simulink model "C_elegans"  (Simulink 7.0)
settings: Solver=ode45  StartTime=0.0  StopTime=10.0  FixedStep=1e-3
undefined symbols (not defined in the file or in its folder): A_n, beta_0M, beta_D, beta_L, c_par, c_per, d_Time, End_Time, eps_hys, F_max_i, G_SR_n, gamma_iD, gamma_iV, I_AVB_D, I_AVB_V, kappa_0M, kappa_D, kappa_L, L_0D_i, L_0L_i, L_min_i, lambda_i, M_num, N_out, N_SR, not_w_NMJ, phi0_vec, R_i, Ri_c_per, S0_nk, tau_M, w_D, w_NMJ, w_V, X_com0
libraries: simulink x1
settings Model: Creator=KRproject  LastModifiedBy=KRproject  SimulationMode=rapid-accelerator
settings OptimizationCC: InlineParams=on  SimCompilerOptimization=On

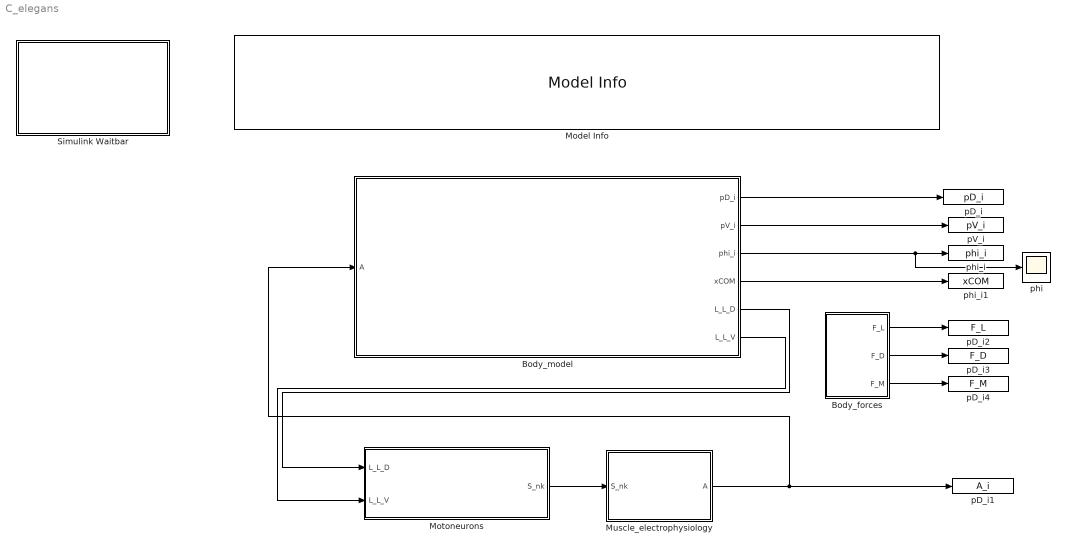
== system C_elegans ==
  Body_forces : Subsystem
  Body_model : Subsystem
      mask Display:
      | image(imread('./pictures/Body_model.png'))
      | port_label('input', 1, 'A')
      | port_label('output', 1, 'pD_i')
      | port_label('output', 2, 'pV_i')
      | port_label('output', 3, 'phi_i')
      | port_label('output', 4, 'xCOM')
      | port_label('output', 5, 'L_L_D')
      | port_label('output', 6, 'L_L_V')
  Model Info : simulink/Model-Wide Utilities/Model Info  SystemSampleTime=-1  InitialBlockCM=None  BlockCM=None  Frame=on  DisplayStringWithTags=|  HorizontalTextAlignment=Center  LeftAlignmentValue=0.5  SourceBlockDiagram=C_elegans  TagMaxNumber=20
      | March 2012
      | C elegans integrated model
      | 
      | ' J. Boyleet al., Gait modulation in C.elegans: an integrated neuromechanical model, Frontiers in Computational Neuroscience, 2012. '
  Motoneurons : Subsystem
  Muscle_electrophysiology : Subsystem
  Simulink Waitbar : Subsystem
      mask Display: image(imread('./pictures/sim_wait.png'))
  pD_i : ToWorkspace  VariableName=pD_i  SampleTime=d_Time  SaveFormat=Array
  pD_i1 : ToWorkspace  VariableName=A_i  SampleTime=d_Time  SaveFormat=Array
  pD_i2 : ToWorkspace  VariableName=F_L  SampleTime=d_Time  SaveFormat=Array
  pD_i3 : ToWorkspace  VariableName=F_D  SampleTime=d_Time  SaveFormat=Array
  pD_i4 : ToWorkspace  VariableName=F_M  SampleTime=d_Time  SaveFormat=Array
  pV_i : ToWorkspace  VariableName=pV_i  SampleTime=d_Time  SaveFormat=Array
  phi : Scope
      settings: TimeRange=10  YMin=-0.75  YMax=3.75
  phi_i : ToWorkspace  VariableName=phi_i  SampleTime=d_Time  SaveFormat=Array
  phi_i1 : ToWorkspace  VariableName=xCOM  SampleTime=d_Time  SaveFormat=Array
  wires:
  Body_model/1(pD_i) -> pD_i/1
  Body_model/2(pV_i) -> pV_i/1
  Body_model/3(phi_i) -> phi_i/1, phi/1
  Body_model/5(L_L_D) -> Motoneurons/1(L_L_D)
  Body_model/6(L_L_V) -> Motoneurons/2(L_L_V)
  Motoneurons/1(S_nk) -> Muscle_electrophysiology/1(S_nk)
  Muscle_electrophysiology/1(A) -> pD_i1/1, Body_model/1(A)
  Body_model/4(xCOM) -> phi_i1/1
  Body_forces/1(F_L) -> pD_i2/1
  Body_forces/2(F_D) -> pD_i3/1
  Body_forces/3(F_M) -> pD_i4/1

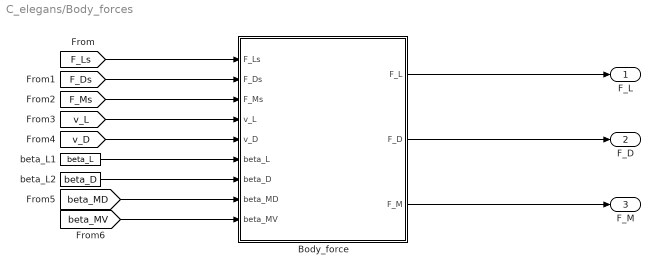
== system C_elegans/Body_forces ==
  Body_force : Stateflow chart
  beta_L1 : Constant  Value=beta_L  OutDataType=sfix(16)  OutScaling=2^0
  beta_L2 : Constant  Value=beta_D  OutDataType=sfix(16)  OutScaling=2^0
  F_L : Outport
  F_D : Outport  Port=2
  F_M : Outport  Port=3
  wires:
  [F_Ls] -> Body_force/1(F_Ls)
  [F_Ds] -> Body_force/2(F_Ds)
  [F_Ms] -> Body_force/3(F_Ms)
  [v_L] -> Body_force/4(v_L)
  [v_D] -> Body_force/5(v_D)
  beta_L1/1 -> Body_force/6(beta_L)
  beta_L2/1 -> Body_force/7(beta_D)
  [beta_MD] -> Body_force/8(beta_MD)
  [beta_MV] -> Body_force/9(beta_MV)
  Body_force/1(F_L) -> F_L/1
  Body_force/2(F_D) -> F_D/1
  Body_force/3(F_M) -> F_M/1

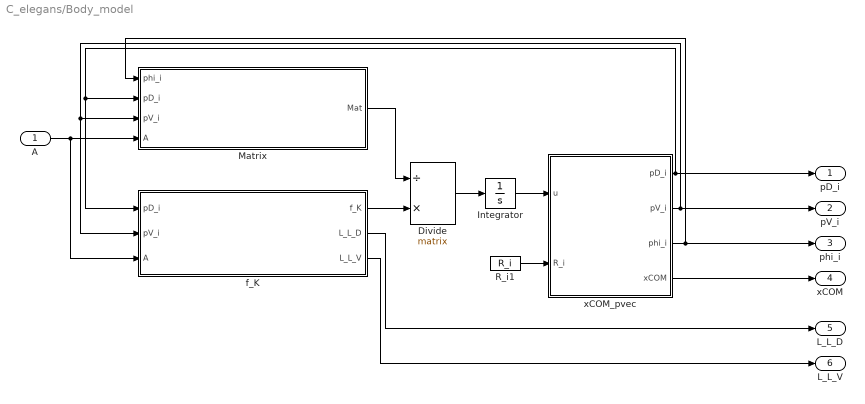
== system C_elegans/Body_model ==
  A : Inport
  Divide : Product  Inputs=/*  Multiplication=Matrix(*)  OutDataType=sfix(16)  OutScaling=2^-10
  Integrator : Integrator  InitialCondition=[ X_com0; phi0_vec]
  Matrix : Subsystem
      mask Display:
      | image(imread('./pictures/Matrix.png'))
      | 
      | port_label('output', 1, 'Mat')
      | port_label('input', 1, 'phi_i')
      | port_label('input', 2, 'pD_i')
      | port_label('input', 3, 'pV_i')
      | port_label('input', 4, 'A')
  R_i1 : Constant  Value=R_i  OutDataType=sfix(16)  OutScaling=2^0
  f_K : Subsystem
      mask Display:
      | image(imread('./pictures/vect.png'))
      | 
      | port_label('output', 1, 'f_K')
      | port_label('output', 2, 'L_L_D')
      | port_label('output', 3, 'L_L_V')
      | 
      | port_label('input', 1, 'pD_i')
      | port_label('input', 2, 'pV_i')
      | port_label('input', 3, 'A')
  xCOM_pvec : Stateflow chart
  pD_i : Outport
  pV_i : Outport  Port=2
  phi_i : Outport  Port=3
  xCOM : Outport  Port=4
  L_L_D : Outport  Port=5
  L_L_V : Outport  Port=6
  wires:
  A/1 -> Matrix/4(A), f_K/3(A)
  Matrix/1(Mat) -> Divide/1
  f_K/1(f_K) -> Divide/2
  Integrator/1 -> xCOM_pvec/1(u)
  R_i1/1 -> xCOM_pvec/2(R_i)
  xCOM_pvec/1(pD_i) -> Matrix/2(pD_i), f_K/1(pD_i), pD_i/1
  xCOM_pvec/2(pV_i) -> Matrix/3(pV_i), f_K/2(pV_i), pV_i/1
  xCOM_pvec/3(phi_i) -> Matrix/1(phi_i), phi_i/1
  f_K/2(L_L_D) -> L_L_D/1
  f_K/3(L_L_V) -> L_L_V/1
  xCOM_pvec/4(xCOM) -> xCOM/1
  Divide/1 -> Integrator/1

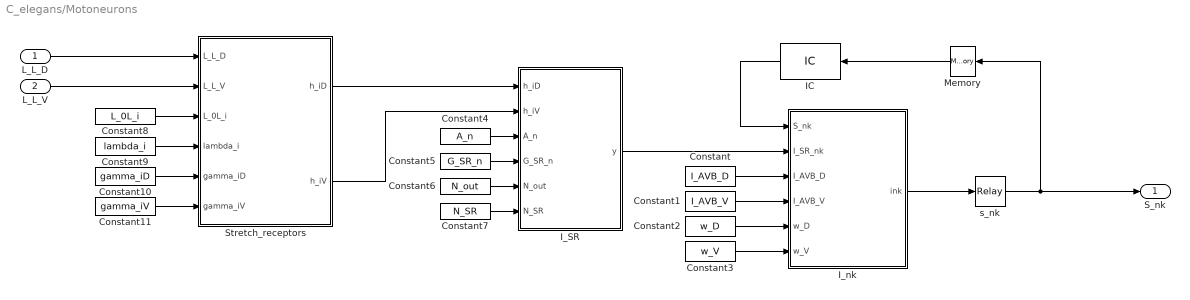
== system C_elegans/Motoneurons ==
  L_L_D : Inport
  L_L_V : Inport  Port=2
  Constant : Constant  Value=I_AVB_D  OutDataType=sfix(16)  OutScaling=2^0
  Constant1 : Constant  Value=I_AVB_V  OutDataType=sfix(16)  OutScaling=2^0
  Constant10 : Constant  Value=gamma_iD  OutDataType=sfix(16)  OutScaling=2^0
  Constant11 : Constant  Value=gamma_iV  OutDataType=sfix(16)  OutScaling=2^0
  Constant2 : Constant  Value=w_D  OutDataType=sfix(16)  OutScaling=2^0
  Constant3 : Constant  Value=w_V  OutDataType=sfix(16)  OutScaling=2^0
  Constant4 : Constant  Value=A_n  OutDataType=sfix(16)  OutScaling=2^0
  Constant5 : Constant  Value=G_SR_n  OutDataType=sfix(16)  OutScaling=2^0
  Constant6 : Constant  Value=N_out  OutDataType=sfix(16)  OutScaling=2^0
  Constant7 : Constant  Value=N_SR  OutDataType=sfix(16)  OutScaling=2^0
  Constant8 : Constant  Value=L_0L_i  OutDataType=sfix(16)  OutScaling=2^0
  Constant9 : Constant  Value=lambda_i  OutDataType=sfix(16)  OutScaling=2^0
  IC : InitialCondition  Orientation=left  Value=S0_nk
  I_SR : Stateflow chart
  I_nk : Stateflow chart
  Memory : Memory  Orientation=left
  Stretch_receptors : Stateflow chart
  s_nk : Relay  OnSwitchValue=0.5*(1 + eps_hys)  OffSwitchValue=0.5*(1 - eps_hys)  OutDataType=sfix(16)  OutScaling=2^0
  S_nk : Outport
  wires:
  s_nk/1 -> S_nk/1, Memory/1
  I_nk/1(ink) -> s_nk/1
  Constant/1 -> I_nk/3(I_AVB_D)
  Constant1/1 -> I_nk/4(I_AVB_V)
  Constant2/1 -> I_nk/5(w_D)
  Constant3/1 -> I_nk/6(w_V)
  IC/1 -> I_nk/1(S_nk)
  I_SR/1(y) -> I_nk/2(I_SR_nk)
  Constant4/1 -> I_SR/3(A_n)
  Constant5/1 -> I_SR/4(G_SR_n)
  Constant6/1 -> I_SR/5(N_out)
  Constant7/1 -> I_SR/6(N_SR)
  Stretch_receptors/1(h_iD) -> I_SR/1(h_iD)
  Stretch_receptors/2(h_iV) -> I_SR/2(h_iV)
  Constant8/1 -> Stretch_receptors/3(L_0L_i)
  Constant9/1 -> Stretch_receptors/4(lambda_i)
  Constant10/1 -> Stretch_receptors/5(gamma_iD)
  Constant11/1 -> Stretch_receptors/6(gamma_iV)
  L_L_D/1 -> Stretch_receptors/1(L_L_D)
  L_L_V/1 -> Stretch_receptors/2(L_L_V)
  Memory/1 -> IC/1

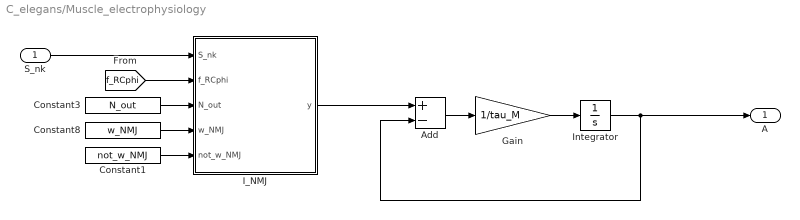
== system C_elegans/Muscle_electrophysiology ==
  S_nk : Inport
  Add : Sum  Inputs=+-  OutDataType=sfix(16)  OutScaling=2^-10
  Constant1 : Constant  Value=not_w_NMJ  OutDataType=sfix(16)  OutScaling=2^0
  Constant3 : Constant  Value=N_out  OutDataType=sfix(16)  OutScaling=2^0
  Constant8 : Constant  Value=w_NMJ  OutDataType=sfix(16)  OutScaling=2^0
  Gain : Gain  Gain=1/tau_M  ParameterDataType=sfix(16)  ParameterScaling=2^0  OutDataType=sfix(16)  OutScaling=2^0
  I_NMJ : Stateflow chart
  Integrator : Integrator  InitialCondition=zeros(2*M_num,1)
  A : Outport
  wires:
  Constant1/1 -> I_NMJ/5(not_w_NMJ)
  Constant8/1 -> I_NMJ/4(w_NMJ)
  I_NMJ/1(y) -> Add/1
  Add/1 -> Gain/1
  Integrator/1 -> Add/2, A/1
  Gain/1 -> Integrator/1
  Constant3/1 -> I_NMJ/3(N_out)
  [f_RCphi] -> I_NMJ/2(f_RCphi)
  S_nk/1 -> I_NMJ/1(S_nk)

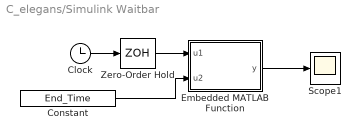
== system C_elegans/Simulink Waitbar ==
  Clock : Clock
  Constant : Constant  Value=End_Time  OutDataType=sfix(16)  OutScaling=2^0
  Embedded MATLAB Function : Stateflow chart
  Scope1 : Scope
      settings: YMin=1  YMax=1  SaveName=ScopeData2
  Zero-Order Hold : ZeroOrderHold
  wires:
  Clock/1 -> Zero-Order Hold/1
  Constant/1 -> Embedded MATLAB Function/2(u2)
  Embedded MATLAB Function/1(y) -> Scope1/1
  Zero-Order Hold/1 -> Embedded MATLAB Function/1(u1)

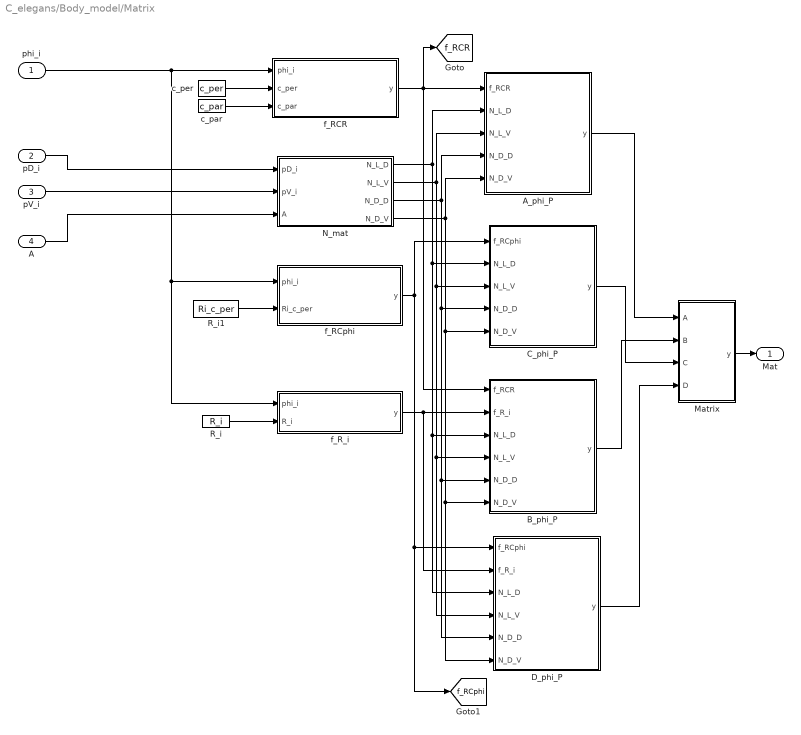
== system C_elegans/Body_model/Matrix ==
  phi_i : Inport
  pD_i : Inport  Port=2
  pV_i : Inport  Port=3
  A : Inport  Port=4
  A_phi_P : Stateflow chart
  B_phi_P : Stateflow chart
  C_phi_P : Stateflow chart
  D_phi_P : Stateflow chart
  Matrix : Stateflow chart
  N_mat : Subsystem
  R_i : Constant  Value=R_i  OutDataType=sfix(16)  OutScaling=2^0
  R_i1 : Constant  Value=Ri_c_per  OutDataType=sfix(16)  OutScaling=2^0
  c_par : Constant  Value=c_par  OutDataType=sfix(16)  OutScaling=2^0
  c_per : Constant  Value=c_per  OutDataType=sfix(16)  OutScaling=2^0
  f_RCR : Stateflow chart
  f_RCphi : Stateflow chart
  f_R_i : Stateflow chart
  Mat : Outport
  tag scope: f_RCR=global, f_RCphi=global
  wires:
  c_per/1 -> f_RCR/2(c_per)
  c_par/1 -> f_RCR/3(c_par)
  f_RCR/1(y) -> A_phi_P/1(f_RCR), B_phi_P/1(f_RCR), [f_RCR]
  N_mat/1(N_L_D) -> A_phi_P/2(N_L_D), C_phi_P/2(N_L_D), B_phi_P/3(N_L_D), D_phi_P/3(N_L_D)
  N_mat/2(N_L_V) -> A_phi_P/3(N_L_V), C_phi_P/3(N_L_V), B_phi_P/4(N_L_V), D_phi_P/4(N_L_V)
  N_mat/3(N_D_D) -> A_phi_P/4(N_D_D), B_phi_P/5(N_D_D), D_phi_P/5(N_D_D), C_phi_P/4(N_D_D)
  N_mat/4(N_D_V) -> A_phi_P/5(N_D_V), B_phi_P/6(N_D_V), D_phi_P/6(N_D_V), C_phi_P/5(N_D_V)
  A_phi_P/1(y) -> Matrix/1(A)
  R_i/1 -> f_R_i/2(R_i)
  f_RCphi/1(y) -> C_phi_P/1(f_RCphi), D_phi_P/1(f_RCphi), [f_RCphi]
  f_R_i/1(y) -> B_phi_P/2(f_R_i), D_phi_P/2(f_R_i)
  C_phi_P/1(y) -> Matrix/3(C)
  B_phi_P/1(y) -> Matrix/2(B)
  D_phi_P/1(y) -> Matrix/4(D)
  phi_i/1 -> f_RCR/1(phi_i), f_R_i/1(phi_i), f_RCphi/1(phi_i)
  pD_i/1 -> N_mat/1(pD_i)
  pV_i/1 -> N_mat/2(pV_i)
  A/1 -> N_mat/3(A)
  Matrix/1(y) -> Mat/1
  R_i1/1 -> f_RCphi/2(Ri_c_per)

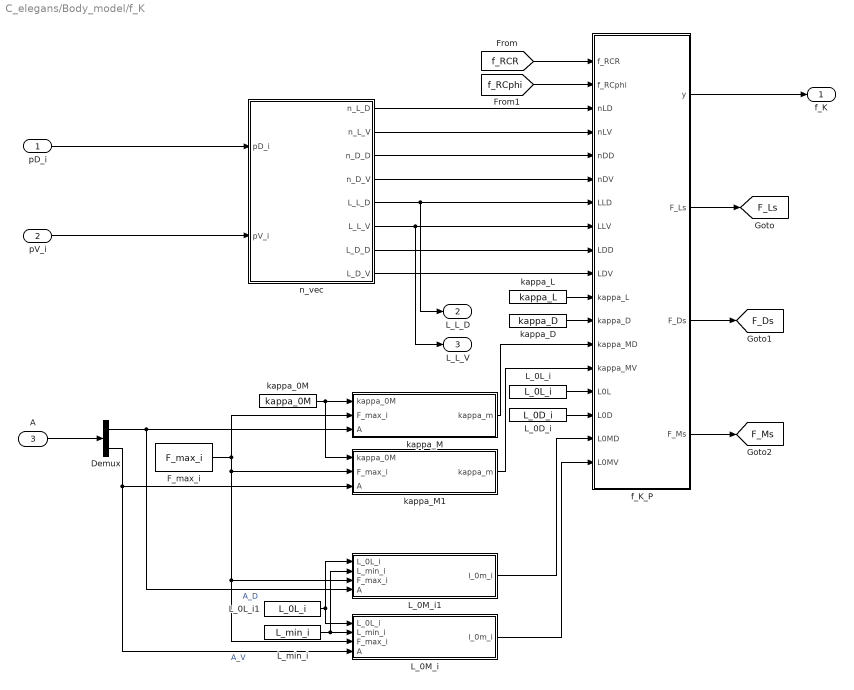
== system C_elegans/Body_model/f_K ==
  pD_i : Inport
  pV_i : Inport  Port=2
  A : Inport  Port=3
  Demux : Demux  Outputs=2
  F_max_i : Constant  Value=F_max_i  OutDataType=sfix(16)  OutScaling=2^0
  L_0D_i : Constant  Value=L_0D_i  OutDataType=sfix(16)  OutScaling=2^0
  L_0L_i : Constant  Value=L_0L_i  OutDataType=sfix(16)  OutScaling=2^0
  L_0L_i1 : Constant  Value=L_0L_i  OutDataType=sfix(16)  OutScaling=2^0
  L_0M_i : Stateflow chart
  L_0M_i1 : Stateflow chart
  L_min_i : Constant  Value=L_min_i  OutDataType=sfix(16)  OutScaling=2^0
  f_K_P : Stateflow chart
  kappa_0M : Constant  Value=kappa_0M  OutDataType=sfix(16)  OutScaling=2^0
  kappa_D : Constant  Value=kappa_D  OutDataType=sfix(16)  OutScaling=2^0
  kappa_L : Constant  Value=kappa_L  OutDataType=sfix(16)  OutScaling=2^0
  kappa_M : Stateflow chart
  kappa_M1 : Stateflow chart
  n_vec : Subsystem
  f_K : Outport
  L_L_D : Outport  Port=2
  L_L_V : Outport  Port=3
  tag scope: F_Ds=global, F_Ls=global, F_Ms=global
  wires:
  n_vec/1(n_L_D) -> f_K_P/3(nLD)
  n_vec/2(n_L_V) -> f_K_P/4(nLV)
  n_vec/3(n_D_D) -> f_K_P/5(nDD)
  n_vec/4(n_D_V) -> f_K_P/6(nDV)
  n_vec/5(L_L_D) -> f_K_P/7(LLD), L_L_D/1
  n_vec/6(L_L_V) -> f_K_P/8(LLV), L_L_V/1
  n_vec/7(L_D_D) -> f_K_P/9(LDD)
  n_vec/8(L_D_V) -> f_K_P/10(LDV)
  L_0L_i/1 -> f_K_P/15(L0L)
  kappa_L/1 -> f_K_P/11(kappa_L)
  L_0D_i/1 -> f_K_P/16(L0D)
  kappa_D/1 -> f_K_P/12(kappa_D)
  kappa_0M/1 -> kappa_M/1(kappa_0M), kappa_M1/1(kappa_0M)
  L_min_i/1 -> L_0M_i/2(L_min_i), L_0M_i1/2(L_min_i)
  F_max_i/1 -> kappa_M/2(F_max_i), kappa_M1/2(F_max_i), L_0M_i/3(F_max_i), L_0M_i1/3(F_max_i)
  kappa_M/1(kappa_m) -> f_K_P/13(kappa_MD)
  L_0M_i/1(l_0m_i) -> f_K_P/18(L0MV)
  pD_i/1 -> n_vec/1(pD_i)
  pV_i/1 -> n_vec/2(pV_i)
  f_K_P/1(y) -> f_K/1
  A/1 -> Demux/1
  Demux/1 -> kappa_M/3(A), L_0M_i1/4(A)  "A_D"
  Demux/2 -> L_0M_i/4(A), kappa_M1/3(A)  "A_V"
  kappa_M1/1(kappa_m) -> f_K_P/14(kappa_MV)
  L_0M_i1/1(l_0m_i) -> f_K_P/17(L0MD)
  L_0L_i1/1 -> L_0M_i/1(L_0L_i), L_0M_i1/1(L_0L_i)
  [f_RCR] -> f_K_P/1(f_RCR)
  [f_RCphi] -> f_K_P/2(f_RCphi)
  f_K_P/2(F_Ls) -> [F_Ls]
  f_K_P/3(F_Ds) -> [F_Ds]
  f_K_P/4(F_Ms) -> [F_Ms]

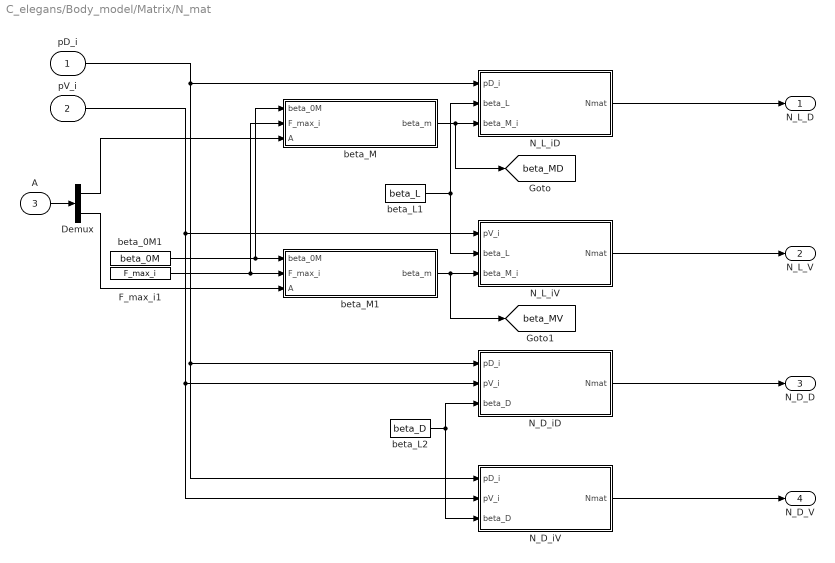
== system C_elegans/Body_model/Matrix/N_mat ==
  pD_i : Inport
  pV_i : Inport  Port=2
  A : Inport  Port=3
  Demux : Demux  Outputs=[M_num,M_num]
  F_max_i1 : Constant  Value=F_max_i  OutDataType=sfix(16)  OutScaling=2^0
  N_D_iD : Stateflow chart
  N_D_iV : Stateflow chart
  N_L_iD : Stateflow chart
  N_L_iV : Stateflow chart
  beta_0M1 : Constant  Value=beta_0M  OutDataType=sfix(16)  OutScaling=2^0
  beta_L1 : Constant  Value=beta_L  OutDataType=sfix(16)  OutScaling=2^0
  beta_L2 : Constant  Value=beta_D  OutDataType=sfix(16)  OutScaling=2^0
  beta_M : Stateflow chart
  beta_M1 : Stateflow chart
  N_L_D : Outport
  N_L_V : Outport  Port=2
  N_D_D : Outport  Port=3
  N_D_V : Outport  Port=4
  tag scope: beta_MD=global, beta_MV=global
  wires:
  beta_M/1(beta_m) -> N_L_iD/3(beta_M_i), [beta_MD]
  Demux/1 -> beta_M/3(A)
  beta_L1/1 -> N_L_iV/2(beta_L), N_L_iD/2(beta_L)
  beta_0M1/1 -> beta_M1/1(beta_0M), beta_M/1(beta_0M)
  F_max_i1/1 -> beta_M1/2(F_max_i), beta_M/2(F_max_i)
  beta_M1/1(beta_m) -> N_L_iV/3(beta_M_i), [beta_MV]
  Demux/2 -> beta_M1/3(A)
  beta_L2/1 -> N_D_iD/3(beta_D), N_D_iV/3(beta_D)
  pD_i/1 -> N_L_iD/1(pD_i), N_D_iD/1(pD_i), N_D_iV/1(pD_i)
  A/1 -> Demux/1
  pV_i/1 -> N_L_iV/1(pV_i), N_D_iD/2(pV_i), N_D_iV/2(pV_i)
  N_L_iD/1(Nmat) -> N_L_D/1
  N_L_iV/1(Nmat) -> N_L_V/1
  N_D_iD/1(Nmat) -> N_D_D/1
  N_D_iV/1(Nmat) -> N_D_V/1

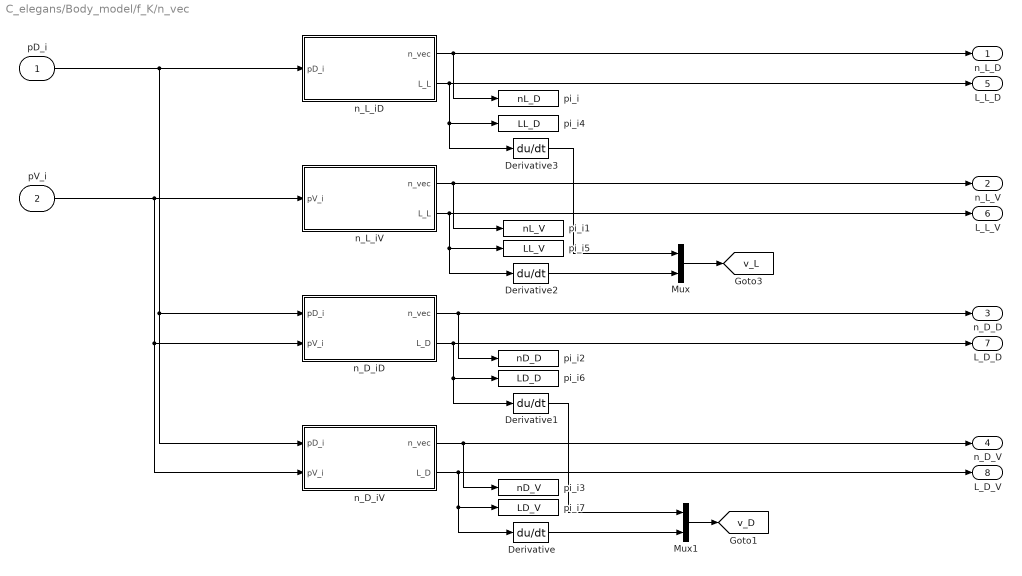
== system C_elegans/Body_model/f_K/n_vec ==
  pD_i : Inport
  pV_i : Inport  Port=2
  Derivative{,1..3} (4 alike) : Derivative
  Mux : Mux  Inputs=2
  Mux1 : Mux  Inputs=2
  n_D_iD : Stateflow chart
  n_D_iV : Stateflow chart
  n_L_iD : Stateflow chart
  n_L_iV : Stateflow chart
  pi_i : ToWorkspace  VariableName=nL_D  SampleTime=d_Time  SaveFormat=Array
  pi_i1 : ToWorkspace  VariableName=nL_V  SampleTime=d_Time  SaveFormat=Array
  pi_i2 : ToWorkspace  VariableName=nD_D  SampleTime=d_Time  SaveFormat=Array
  pi_i3 : ToWorkspace  VariableName=nD_V  SampleTime=d_Time  SaveFormat=Array
  pi_i4 : ToWorkspace  VariableName=LL_D  SampleTime=d_Time  SaveFormat=Array
  pi_i5 : ToWorkspace  VariableName=LL_V  SampleTime=d_Time  SaveFormat=Array
  pi_i6 : ToWorkspace  VariableName=LD_D  SampleTime=d_Time  SaveFormat=Array
  pi_i7 : ToWorkspace  VariableName=LD_V  SampleTime=d_Time  SaveFormat=Array
  n_L_D : Outport
  n_L_V : Outport  Port=2
  n_D_D : Outport  Port=3
  n_D_V : Outport  Port=4
  L_L_D : Outport  Port=5
  L_L_V : Outport  Port=6
  L_D_D : Outport  Port=7
  L_D_V : Outport  Port=8
  tag scope: v_D=global, v_L=global
  wires:
  pD_i/1 -> n_L_iD/1(pD_i), n_D_iD/1(pD_i), n_D_iV/1(pD_i)
  pV_i/1 -> n_L_iV/1(pV_i), n_D_iD/2(pV_i), n_D_iV/2(pV_i)
  n_L_iD/1(n_vec) -> n_L_D/1, pi_i/1
  n_L_iV/1(n_vec) -> n_L_V/1, pi_i1/1
  n_D_iD/1(n_vec) -> n_D_D/1, pi_i2/1
  n_D_iV/1(n_vec) -> n_D_V/1, pi_i3/1
  n_L_iD/2(L_L) -> L_L_D/1, pi_i4/1, Derivative3/1
  n_L_iV/2(L_L) -> L_L_V/1, pi_i5/1, Derivative2/1
  n_D_iD/2(L_D) -> L_D_D/1, pi_i6/1, Derivative1/1
  n_D_iV/2(L_D) -> L_D_V/1, pi_i7/1, Derivative/1
  Mux1/1 -> [v_D]
  Mux/1 -> [v_L]
  Derivative/1 -> Mux1/2
  Derivative2/1 -> Mux/2
  Derivative3/1 -> Mux/1
  Derivative1/1 -> Mux1/1

== matlab function Body_model/f_K/kappa_M1 ==
  data: kappa_0M input inherited; kappa_m output inherited; F_max_i input inherited; A input inherited
function kappa_m = kappa_M( kappa_0M, F_max_i, A)
% This block supports the Embedded MATLAB subset.
% See the help menu for details. 

sig_A = A.*( 0 < A & A < 1) + (1 <= A);

kappa_m = kappa_0M.*F_max_i.*sig_A;

== matlab function Body_model/f_K/L_0M_i1 ==
  data: L_0L_i input inherited; L_min_i input inherited; l_0m_i output inherited; F_max_i input inherited; A input inherited
function l_0m_i = L_0M_i( L_0L_i, L_min_i, F_max_i, A)
% This block supports the Embedded MATLAB subset.
% See the help menu for details. 

sig_A = A.*( 0 < A & A < 1) + (1 <= A);

l_0m_i = L_0L_i - F_max_i.*sig_A.*(L_0L_i - L_min_i);

== matlab function Motoneurons/I_nk ==
  data: S_nk input inherited; I_SR_nk input inherited; ink output inherited; I_AVB_D input inherited; I_AVB_V input inherited; w_D input inherited; w_V input inherited
function ink = I_nk( S_nk, I_SR_nk, I_AVB_D, I_AVB_V, w_D, w_V)
% This block supports the Embedded MATLAB subset.
% See the help menu for details. 

N_num = length( S_nk)/2;

S_nD = S_nk(1:N_num);
S_nV = S_nk(N_num+1:end);

I_SR_nD = I_SR_nk(1:N_num);
I_SR_nV = I_SR_nk(N_num+1:end);


ink = 0*S_nk;
ink(1:N_num) = I_AVB_D + I_SR_nD + w_D*S_nV;
ink(N_num+1:end) = I_AVB_V + I_SR_nV + w_V*S_nD;

== matlab function Motoneurons/I_SR ==
  data: h_iD input inherited; h_iV input inherited; y output inherited; A_n input inherited; G_SR_n input inherited; N_out input inherited; N_SR input inherited
function y = I_SR( h_iD, h_iV, A_n, G_SR_n, N_out, N_SR)
% This block supports the Embedded MATLAB subset.
% See the help menu for details. 

N_num = length( A_n);
M_num = length( h_iD);

H_iD = 0*A_n;
H_iV = 0*A_n;
for n = 1:N_num 
    
    s_end = min( M_num, N_SR + (n - 1)*N_out);
    for m = 1:M_num
        
        H_iD(n) = H_iD(n) + h_iD(m).*( (n-1)*N_out+1 <= m & m <= s_end);
        H_iV(n) = H_iV(n) + h_iV(m).*( (n-1)*N_out+1 <= m & m <= s_end);
    end
end

y = repmat( A_n.*G_SR_n, 2, 1).*[ H_iD; 
                                  H_iV];

== matlab function Motoneurons/Stretch_receptors ==
  data: L_L_D input inherited; h_iD output inherited; L_L_V input inherited; L_0L_i input inherited; lambda_i input inherited; gamma_iD input inherited; gamma_iV input inherited; h_iV output inherited
function [h_iD,h_iV] = h_ik( L_L_D, L_L_V, L_0L_i, lambda_i, gamma_iD, gamma_iV)
% This block supports the Embedded MATLAB subset.
% See the help menu for details. 

h_iD = lambda_i.*( gamma_iD(1)*(L_L_D - L_0L_i)./L_0L_i.*(L_L_D > L_0L_i) ...
                  + gamma_iD(2)*(L_L_D - L_0L_i)./L_0L_i.*(L_L_D <= L_0L_i) );
h_iV = lambda_i*gamma_iV.*(L_L_V - L_0L_i)./L_0L_i;

== matlab function Simulink Waitbar/Embedded MATLAB Function ==
  data: u1 input inherited; y output inherited; u2 input inherited
function y = fcn(u1, u2)
% This block supports an embeddable subset of the MATLAB language.
% See the help menu for details. 

eml.extrinsic('waitbar')

waitbar(u1/u2)
y = 1;

== matlab function Muscle_electrophysiology/I_NMJ ==
  data: S_nk input inherited; f_RCphi input inherited; N_out input inherited; y output inherited; w_NMJ input inherited; not_w_NMJ input inherited
function y = I_NMJ( S_nk, f_RCphi, N_out, w_NMJ, not_w_NMJ)
% This block supports the Embedded MATLAB subset.
% See the help menu for details. 

N_num = length( S_nk)/2;

S_nD = S_nk(1:N_num);
S_nV = S_nk(N_num+1:end);

M_num = size( f_RCphi, 1) - 1;
zero_vec = 0*f_RCphi(1:end-1,1);
i_NMJ_D = zero_vec;
i_NMJ_V = zero_vec;
for i=1:M_num
    
    n = ceil( i/N_out);
    
    i_NMJ_D(i) = w_NMJ(n)*S_nD(n) + not_w_NMJ(n)*S_nV(n);
    i_NMJ_V(i) = w_NMJ(n)*S_nV(n) + not_w_NMJ(n)*S_nD(n);
end

y = [ i_NMJ_D;
      i_NMJ_V];

== matlab function Body_forces/Body_force ==
  data: F_Ls input inherited; F_L output inherited; F_Ds input inherited; F_Ms input inherited; v_L input inherited; v_D input inherited; beta_L input inherited; beta_D input inherited; beta_MD input inherited; beta_MV input inherited; F_D output inherited; F_M output inherited
function [ F_L, F_D, F_M] = Body_forces( F_Ls, F_Ds, F_Ms, v_L, v_D, beta_L, beta_D, beta_MD, beta_MV)
% This block supports the Embedded MATLAB subset.
% See the help menu for details. 

M_num_p1 = length( F_Ls)/2;

F_Ldamp = -beta_L*v_L;
F_Ddamp = -beta_D*v_D;
F_Mdamp = -[ beta_MD; beta_MV].*v_L;

F_L = F_Ls + F_Ldamp;
F_D = F_Ds + F_Ddamp;
F_M = F_Ms + F_Mdamp;

== matlab function Body_model/Matrix/f_RCR ==
  data: phi_i input inherited; y output inherited; c_per input inherited; c_par input inherited
function y = f_RCR( phi_i, c_per, c_par)
% This block supports the Embedded MATLAB subset.
% See the help menu for details. 

M_num_p1 = length( phi_i);

h_sin_mat = kron( sin( phi_i), [1 1].');
h_cos_mat = zeros( 2*M_num_p1-1, 1);
h_cos_mat(1:2:end) = cos( phi_i);

R_mat = diag( h_sin_mat) + diag( h_cos_mat, 1) - diag( h_cos_mat, -1);
CC_mat = diag( repmat( [c_per^-1 c_par^-1].', M_num_p1, 1) );

y = R_mat*CC_mat*R_mat.';

== matlab function Body_model/Matrix/N_mat/N_L_iD ==
  data: pD_i input inherited; Nmat output inherited; beta_L input inherited; beta_M_i input inherited
function Nmat = N_L_iD( pD_i, beta_L, beta_M_i)
% This block supports the Embedded MATLAB subset.
% See the help menu for details. 

M_num_p1 = size( pD_i, 1);

L_L = sqrt( (pD_i(2:end,1) - pD_i(1:end-1,1)).^2 + (pD_i(2:end,2) - pD_i(1:end-1,2)).^2 );

n_vec = ( pD_i(1:end-1,:) - pD_i(2:end,:) )./(L_L*[1 1]);

n_vec2 = reshape( n_vec.', [], 1);

Nmat = zeros(2*M_num_p1);
for ii = 1:M_num_p1-1
    ii_vec = [2*ii-1 2*ii];
    Nmat(ii_vec,ii_vec) = (beta_L + beta_M_i(ii))*n_vec2(ii_vec)*n_vec2(ii_vec).';
end

== matlab function Body_model/Matrix/N_mat/N_L_iV ==
  data: pV_i input inherited; Nmat output inherited; beta_L input inherited; beta_M_i input inherited
function Nmat = N_L_iV( pV_i, beta_L, beta_M_i)
% This block supports the Embedded MATLAB subset.
% See the help menu for details. 

M_num_p1 = size( pV_i, 1);

L_L = sqrt( (pV_i(2:end,1) - pV_i(1:end-1,1)).^2 + (pV_i(2:end,2) - pV_i(1:end-1,2)).^2 );

n_vec = ( pV_i(1:end-1,:) - pV_i(2:end,:) )./(L_L*[1 1]);

n_vec2 = reshape( n_vec.', [], 1);

Nmat = zeros(2*M_num_p1);
for ii = 1:M_num_p1-1
    ii_vec = [2*ii-1 2*ii];
    Nmat(ii_vec,ii_vec) = (beta_L + beta_M_i(ii))*n_vec2(ii_vec)*n_vec2(ii_vec).';
end

== matlab function Body_model/Matrix/N_mat/beta_M ==
  data: beta_0M input inherited; beta_m output inherited; F_max_i input inherited; A input inherited
function beta_m = beta_M( beta_0M, F_max_i, A)
% This block supports the Embedded MATLAB subset.
% See the help menu for details. 

sig_A = A.*( 0 < A & A < 1) + (1 <= A);

beta_m = beta_0M.*F_max_i.*sig_A;

== matlab function Body_model/Matrix/N_mat/beta_M1 ==
  data: beta_0M input inherited; beta_m output inherited; F_max_i input inherited; A input inherited
function beta_m = beta_M( beta_0M, F_max_i, A)
% This block supports the Embedded MATLAB subset.
% See the help menu for details. 

sig_A = A.*( 0 < A & A < 1) + (1 <= A);

beta_m = beta_0M.*F_max_i.*sig_A;

== matlab function Body_model/Matrix/A_phi_P ==
  data: f_RCR input inherited; y output inherited; N_L_D input inherited; N_L_V input inherited; N_D_D input inherited; N_D_V input inherited
function y = A_phi_P( f_RCR, N_L_D, N_L_V, N_D_D, N_D_V)
% This block supports the Embedded MATLAB subset.
% See the help menu for details. 

M_num_p1 = size( f_RCR, 1)/2;

% zero_mat = zeros(2*M_num_p1);
zero_mat = 0*N_L_D;
NLD_im1 = zero_mat;
NLV_im1 = zero_mat;
NDD_im1 = zero_mat;
NDV_im1 = zero_mat;

NLD_im1(3:end,3:end) = N_L_D(1:end-2,1:end-2);
NLV_im1(3:end,3:end) = N_L_V(1:end-2,1:end-2);
NDD_im1(3:end,3:end) = N_D_D(1:end-2,1:end-2);
NDV_im1(3:end,3:end) = N_D_V(1:end-2,1:end-2);

NLD_i = N_L_D;
NLV_i = N_L_V;
NDD_i = N_D_D;
NDV_i = N_D_V;



a_im1 = -f_RCR*( NLD_im1 + NLV_im1 + NDV_im1 + NDD_im1 );
A_im1 = zero_mat;
A_im1(3:end,1:end-2) = a_im1(3:end,3:end);


a_i = eye(2*M_num_p1) + f_RCR*( NLD_i + NLV_i + NLD_im1 + NLV_im1...
                    + NDD_i + NDV_i + NDV_im1 + NDD_im1 );
A_i = a_i;
                

a_ip1 = -f_RCR*( NLD_i + NLV_i + NDD_i + NDV_i );
A_ip1 = zero_mat;
A_ip1(1:end-2,3:end) = a_ip1(1:end-2,1:end-2);


y = A_im1 + A_i + A_ip1;

== matlab function Body_model/Matrix/f_RCphi ==
  data: phi_i input inherited; y output inherited; Ri_c_per input inherited
function y = f_RCphi( phi_i, Ri_c_per)
% This block supports the Embedded MATLAB subset.
% See the help menu for details. 

M_num_p1 = length( phi_i);

zero_mat = zeros( M_num_p1, 2*M_num_p1);
h_sin_mat = zero_mat;
h_sin_mat(:,1:2:end-1) = diag( sin( phi_i));
h_cos_mat = zero_mat;
h_cos_mat(:,2:2:end) = diag( cos( phi_i));

R_mat = h_sin_mat - h_cos_mat;

y = ( 1./Ri_c_per*ones(1,2*M_num_p1) ).*R_mat;

== matlab function Body_model/Matrix/N_mat/N_D_iD ==
  data: pD_i input inherited; pV_i input inherited; Nmat output inherited; beta_D input inherited
function Nmat = N_D_iD( pD_i, pV_i, beta_D)
% This block supports the Embedded MATLAB subset.
% See the help menu for details. 

M_num_p1 = size( pD_i, 1);

L_D = sqrt( (pV_i(2:end,1) - pD_i(1:end-1,1)).^2 + (pV_i(2:end,2) - pD_i(1:end-1,2)).^2 );

n_vec = ( pD_i(1:end-1,:) - pV_i(2:end,:) )./(L_D*[1 1]);

n_vec2 = reshape( n_vec.', [], 1);

Nmat = zeros(2*M_num_p1);
for ii = 1:M_num_p1-1
    ii_vec = [2*ii-1 2*ii];
    Nmat(ii_vec,ii_vec) = beta_D*n_vec2(ii_vec)*n_vec2(ii_vec).';
end

== matlab function Body_model/Matrix/N_mat/N_D_iV ==
  data: pD_i input inherited; pV_i input inherited; Nmat output inherited; beta_D input inherited
function Nmat = N_D_iV( pD_i, pV_i, beta_D)
% This block supports the Embedded MATLAB subset.
% See the help menu for details. 

M_num_p1 = size( pD_i, 1);

L_D = sqrt( (pD_i(2:end,1) - pV_i(1:end-1,1)).^2 + (pD_i(2:end,2) - pV_i(1:end-1,2)).^2 );

n_vec = ( pV_i(1:end-1,:) - pD_i(2:end,:) )./(L_D*[1 1]);

n_vec2 = reshape( n_vec.', [], 1);

Nmat = zeros(2*M_num_p1);
for ii = 1:M_num_p1-1
    ii_vec = [2*ii-1 2*ii];
    Nmat(ii_vec,ii_vec) = beta_D*n_vec2(ii_vec)*n_vec2(ii_vec).';
end

== matlab function Body_model/Matrix/C_phi_P ==
  data: f_RCphi input inherited; y output inherited; N_L_D input inherited; N_L_V input inherited; N_D_D input inherited; N_D_V input inherited
function y = C_phi_P( f_RCphi, N_L_D, N_L_V, N_D_D, N_D_V)
% This block supports the Embedded MATLAB subset.
% See the help menu for details. 

M_num_p1 = size( f_RCphi, 1);

% zero_mat = zeros(2*M_num_p1);
zero_mat = 0*N_L_D;
NLD_im1 = zero_mat;
NLV_im1 = zero_mat;
NDD_im1 = zero_mat;
NDV_im1 = zero_mat;

NLD_im1(3:end,3:end) = N_L_D(1:end-2,1:end-2);
NLV_im1(3:end,3:end) = N_L_V(1:end-2,1:end-2);
NDD_im1(3:end,3:end) = N_D_D(1:end-2,1:end-2);
NDV_im1(3:end,3:end) = N_D_V(1:end-2,1:end-2);

NLD_i = N_L_D;
NLV_i = N_L_V;
NDD_i = N_D_D;
NDV_i = N_D_V;


% zero_mat2 = zeros(M_num_p1,2*M_num_p1);
zero_mat2 = 0*f_RCphi;
c_im1 = f_RCphi*( NLD_im1 - NLV_im1 + NDV_im1 - NDD_im1 );
C_im1 = zero_mat2;
C_im1(2:end,1:end-2) = c_im1(2:end,3:end);

c_i = -f_RCphi*( NLD_i - NLV_i + NLD_im1 - NLV_im1...
                    + NDD_i - NDV_i + NDV_im1 - NDD_im1 );
C_i = c_i;

                
c_ip1 = f_RCphi*( NLD_i - NLV_i + NDD_i - NDV_i );
C_ip1 = zero_mat2;
C_ip1(1:end-1,3:end) = c_ip1(1:end-1,1:end-2);


y = C_im1 + C_i + C_ip1;

== matlab function Body_model/Matrix/B_phi_P ==
  data: f_RCR input inherited; f_R_i input inherited; y output inherited; N_L_D input inherited; N_L_V input inherited; N_D_D input inherited; N_D_V input inherited
function y = B_phi_P( f_RCR, f_R_i, N_L_D, N_L_V, N_D_D, N_D_V)
% This block supports the Embedded MATLAB subset.
% See the help menu for details. 

M_num_p1 = size( f_RCR, 1)/2;

% zero_mat = zeros(2*M_num_p1);
zero_mat = 0*N_L_D;
NLD_im1 = zero_mat;
NLV_im1 = zero_mat;
NDD_im1 = zero_mat;
NDV_im1 = zero_mat;

NLD_im1(3:end,3:end) = N_L_D(1:end-2,1:end-2);
NLV_im1(3:end,3:end) = N_L_V(1:end-2,1:end-2);
NDD_im1(3:end,3:end) = N_D_D(1:end-2,1:end-2);
NDV_im1(3:end,3:end) = N_D_V(1:end-2,1:end-2);

NLD_i = N_L_D;
NLV_i = N_L_V;
NDD_i = N_D_D;
NDV_i = N_D_V;

% zero_mat2 = zeros(2*M_num_p1,M_num_p1);
zero_mat2 = 0*f_R_i;
f_R_im1 = zero_mat2;
f_R_im1(3:end,2:end) = f_R_i(1:end-2,1:end-1);
f_R_ip1 = zero_mat2;
f_R_ip1(1:end-2,1:end-1) = f_R_i(3:end,2:end);


b_im1 = -f_RCR*( NLD_im1 - NLV_im1 - NDV_im1 + NDD_im1 )*f_R_im1;
B_im1 = zero_mat2;
B_im1(3:end,1:end-1) = b_im1(3:end,2:end);

b_i = f_RCR*( NLD_i - NLV_i + NLD_im1 - NLV_im1...
                    + NDD_i - NDV_i + NDV_im1 - NDD_im1 )*f_R_i;
B_i = b_i;

                
b_ip1 = -f_RCR*( NLD_i - NLV_i - NDD_i + NDV_i )*f_R_ip1;
B_ip1 = zero_mat2;
B_ip1(1:end-2,2:end) = b_ip1(1:end-2,1:end-1);


y = B_im1 + B_i + B_ip1;

== matlab function Body_model/Matrix/f_R_i ==
  data: phi_i input inherited; y output inherited; R_i input inherited
function y = f_R_i( phi_i, R_i)
% This block supports the Embedded MATLAB subset.
% See the help menu for details. 

M_num_p1 = length( phi_i);

zero_mat = zeros( M_num_p1, 2*M_num_p1);
h_sin_mat = zero_mat;
h_sin_mat(:,1:2:end-1) = diag( sin( phi_i));
h_cos_mat = zero_mat;
h_cos_mat(:,2:2:end) = diag( cos( phi_i));

R_mat = -h_sin_mat + h_cos_mat;

y = ( ones(2*M_num_p1,1)*R_i.' ).*R_mat.';

== matlab function Body_model/Matrix/D_phi_P ==
  data: f_RCphi input inherited; f_R_i input inherited; y output inherited; N_L_D input inherited; N_L_V input inherited; N_D_D input inherited; N_D_V input inherited
function y = D_phi_P( f_RCphi, f_R_i, N_L_D, N_L_V, N_D_D, N_D_V)
% This block supports the Embedded MATLAB subset.
% See the help menu for details. 

M_num_p1 = size( f_RCphi, 1);

% zero_mat = zeros(2*M_num_p1);
zero_mat = 0*N_L_D;
NLD_im1 = zero_mat;
NLV_im1 = zero_mat;
NDD_im1 = zero_mat;
NDV_im1 = zero_mat;

NLD_im1(3:end,3:end) = N_L_D(1:end-2,1:end-2);
NLV_im1(3:end,3:end) = N_L_V(1:end-2,1:end-2);
NDD_im1(3:end,3:end) = N_D_D(1:end-2,1:end-2);
NDV_im1(3:end,3:end) = N_D_V(1:end-2,1:end-2);

NLD_i = N_L_D;
NLV_i = N_L_V;
NDD_i = N_D_D;
NDV_i = N_D_V;

% zero_mat2 = zeros(2*M_num_p1,M_num_p1);
zero_mat2 = 0*f_R_i;
f_R_im1 = zero_mat2;
f_R_im1(3:end,2:end) = f_R_i(1:end-2,1:end-1);
f_R_ip1 = zero_mat2;
f_R_ip1(1:end-2,1:end-1) = f_R_i(3:end,2:end);


% zero_mat3 = zeros(M_num_p1);
zero_mat3 = 0*N_L_D(1:end/2,1:end/2);
d_im1 = f_RCphi*( NLD_im1 + NLV_im1 - NDV_im1 - NDD_im1 )*f_R_im1;
D_im1 = zero_mat3;
D_im1(2:end,1:end-1) = d_im1(2:end,2:end);

d_i = eye(M_num_p1) - f_RCphi*( NLD_i + NLV_i + NLD_im1 + NLV_im1...
                                + NDD_i + NDV_i + NDV_im1 + NDD_im1 )*f_R_i;
D_i = d_i;
                            
                
d_ip1 = f_RCphi*( NLD_i + NLV_i - NDD_i - NDV_i )*f_R_ip1;
D_ip1 = zero_mat3;
D_ip1(1:end-1,2:end) = d_ip1(1:end-1,1:end-1);


y = D_im1 + D_i + D_ip1;

== matlab function Body_model/Matrix/Matrix ==
  data: A input inherited; y output inherited; B input inherited; C input inherited; D input inherited
function y = Matrix( A, B, C, D)
% This block supports the Embedded MATLAB subset.
% See the help menu for details. 

y = [ A B;
      C D];

== matlab function Body_model/f_K/n_vec/n_D_iD ==
  data: pD_i input inherited; pV_i input inherited; n_vec output inherited; L_D output inherited
function [n_vec,L_D] = n_D_iD( pD_i, pV_i)
% This block supports the Embedded MATLAB subset.
% See the help menu for details. 


L_D = sqrt( (pV_i(2:end,1) - pD_i(1:end-1,1)).^2 + (pV_i(2:end,2) - pD_i(1:end-1,2)).^2 );

n_vec = ( pD_i(1:end-1,:) - pV_i(2:end,:) )./(L_D*[1 1]);

== matlab function Body_model/f_K/n_vec/n_D_iV ==
  data: pD_i input inherited; pV_i input inherited; n_vec output inherited; L_D output inherited
function [n_vec,L_D] = n_D_iV( pD_i, pV_i)
% This block supports the Embedded MATLAB subset.
% See the help menu for details. 



L_D = sqrt( (pD_i(2:end,1) - pV_i(1:end-1,1)).^2 + (pD_i(2:end,2) - pV_i(1:end-1,2)).^2 );

n_vec = ( pV_i(1:end-1,:) - pD_i(2:end,:) )./(L_D*[1 1]);

== matlab function Body_model/f_K/n_vec/n_L_iD ==
  data: pD_i input inherited; n_vec output inherited; L_L output inherited
function [n_vec,L_L] = n_L_iD( pD_i)
% This block supports the Embedded MATLAB subset.
% See the help menu for details. 



L_L = sqrt( (pD_i(2:end,1) - pD_i(1:end-1,1)).^2 + (pD_i(2:end,2) - pD_i(1:end-1,2)).^2 );

n_vec = ( pD_i(1:end-1,:) - pD_i(2:end,:) )./(L_L*[1 1]);

== matlab function Body_model/f_K/n_vec/n_L_iV ==
  data: pV_i input inherited; n_vec output inherited; L_L output inherited
function [n_vec,L_L] = n_L_iV( pV_i)
% This block supports the Embedded MATLAB subset.
% See the help menu for details. 



L_L = sqrt( (pV_i(2:end,1) - pV_i(1:end-1,1)).^2 + (pV_i(2:end,2) - pV_i(1:end-1,2)).^2 );

n_vec = ( pV_i(1:end-1,:) - pV_i(2:end,:) )./(L_L*[1 1]);

== matlab function Body_model/f_K/f_K_P ==
  data: f_RCR input inherited; f_RCphi input inherited; nLD input inherited; nLV input inherited; nDD input inherited; nDV input inherited; LLD input inherited; y output inherited; LLV input inherited; LDD input inherited; LDV input inherited; kappa_L input inherited; kappa_D input inherited; kappa_MD input inherited; kappa_MV input inherited; L0L input inherited; L0D input inherited; L0MD input inherited; L0MV input inherited; F_Ls output inherited; F_Ds output inherited; F_Ms output inherited
function [y, F_Ls, F_Ds, F_Ms] = f_K_P( f_RCR, f_RCphi, nLD, nLV, nDD, nDV, LLD, LLV, LDD, LDV, kappa_L, kappa_D, kappa_MD, kappa_MV, L0L, L0D, L0MD, L0MV)
% This block supports the Embedded MATLAB subset.
% See the help menu for details. 

M_num_p1 = size( f_RCR, 1)/2;

%% 復元力の大きさ
KLD = kappa_L*( (L0L - LLD) + 2*(L0L - LLD).^4.*(LLD >= L0L) );
KLV = kappa_L*( (L0L - LLV) + 2*(L0L - LLV).^4.*(LLV >= L0L) );
F_Ls = [ KLD;
         KLV];

KDD = kappa_D*(L0D - LDD);
KDV = kappa_D*(L0D - LDV);
F_Ds = [ KDD;
         KDV];

KMD = kappa_MD.*(L0MD - LLD);
KMV = kappa_MV.*(L0MV - LLV);
F_Ms = [ KMD;
         KMV];

%% 方向ベクトル
nLD2 = reshape( nLD.', [], 1);
nLV2 = reshape( nLV.', [], 1);
nDD2 = reshape( nDD.', [], 1);
nDV2 = reshape( nDV.', [], 1);

%% 復元力
% zero_vec = zeros(2*M_num_p1,1);
zero_vec = 0*f_RCR(:,1);
KLD_n_i = zero_vec;
KLV_n_i = zero_vec;
KDD_n_i = zero_vec;
KDV_n_i = zero_vec;
KMD_n_i = zero_vec;
KMV_n_i = zero_vec;

KLD_n_i(1:end-2) = kron( KLD, [1 1].').*nLD2;
KLV_n_i(1:end-2) = kron( KLV, [1 1].').*nLV2;
KDD_n_i(1:end-2) = kron( KDD, [1 1].').*nDD2;
KDV_n_i(1:end-2) = kron( KDV, [1 1].').*nDV2;
KMD_n_i(1:end-2) = kron( KMD, [1 1].').*nLD2;
KMV_n_i(1:end-2) = kron( KMV, [1 1].').*nLV2;


KLD_n_im1 = zero_vec;
KLV_n_im1 = zero_vec;
KDD_n_im1 = zero_vec;
KDV_n_im1 = zero_vec;
KMD_n_im1 = zero_vec;
KMV_n_im1 = zero_vec;

KLD_n_im1(3:end) = KLD_n_i(1:end-2);
KLV_n_im1(3:end) = KLV_n_i(1:end-2);
KDD_n_im1(3:end) = KDD_n_i(1:end-2);
KDV_n_im1(3:end) = KDV_n_i(1:end-2);
KMD_n_im1(3:end) = KMD_n_i(1:end-2);
KMV_n_im1(3:end) = KMV_n_i(1:end-2);


f_K_P1 = f_RCR*( KLD_n_i - KLD_n_im1 + KDD_n_i - KDV_n_im1 + KMD_n_i - KMD_n_im1 ...
            + KLV_n_i - KLV_n_im1 + KDV_n_i - KDD_n_im1 + KMV_n_i - KMV_n_im1 );
        
f_K_P2 = -f_RCphi*( KLD_n_i - KLD_n_im1 + KDD_n_i - KDV_n_im1 + KMD_n_i - KMD_n_im1 ...
            - KLV_n_i + KLV_n_im1 - KDV_n_i + KDD_n_im1 - KMV_n_i + KMV_n_im1 );
        
y = [ f_K_P1; 
      f_K_P2];

== matlab function Body_model/f_K/L_0M_i ==
  data: L_0L_i input inherited; L_min_i input inherited; l_0m_i output inherited; F_max_i input inherited; A input inherited
function l_0m_i = L_0M_i( L_0L_i, L_min_i, F_max_i, A)
% This block supports the Embedded MATLAB subset.
% See the help menu for details. 

sig_A = A.*( 0 < A & A < 1) + (1 <= A);

l_0m_i = L_0L_i - F_max_i.*sig_A.*(L_0L_i - L_min_i);

== matlab function Body_model/f_K/kappa_M ==
  data: kappa_0M input inherited; kappa_m output inherited; F_max_i input inherited; A input inherited
function kappa_m = kappa_M( kappa_0M, F_max_i, A)
% This block supports the Embedded MATLAB subset.
% See the help menu for details. 

sig_A = A.*( 0 < A & A < 1) + (1 <= A);

kappa_m = kappa_0M.*F_max_i.*sig_A;

== matlab function Body_model/xCOM_pvec ==
  data: u input inherited; pD_i output inherited; R_i input inherited; pV_i output inherited; phi_i output inherited; xCOM output inherited
function [pD_i,pV_i, phi_i, xCOM] = xCOM_pvec( u, R_i)
% This block supports the Embedded MATLAB subset.
% See the help menu for details. 

M_num_p1 = length( R_i);

xCOM = u(1:2*M_num_p1);
phi_i = u(2*M_num_p1+1:end);

cos_sin_vec = 0*xCOM;
cos_sin_vec(1:2:end-1) = cos( phi_i);
cos_sin_vec(2:2:end) = sin( phi_i);


dx_v = kron( R_i, [1 1].').*cos_sin_vec;
pD = xCOM + dx_v;
pV = xCOM - dx_v;

pD_i = reshape( pD, 2, []).';
pV_i = reshape( pV, 2, []).';
